simulink model "s_function_model"  (R2021b)
settings: Solver=FixedStepAuto  StartTime=0.0  StopTime=10.0  RelTol=1e-3
settings Model: Creator=krzysztof  LastModifiedBy=krzysztof
settings SolverCC: ZeroCrossControl=DisableAll
settings DataIOCC: SaveOutput=off  SaveTime=off
settings OptimizationCC: BlockReduction=off  DefaultParameterBehavior=Inlined

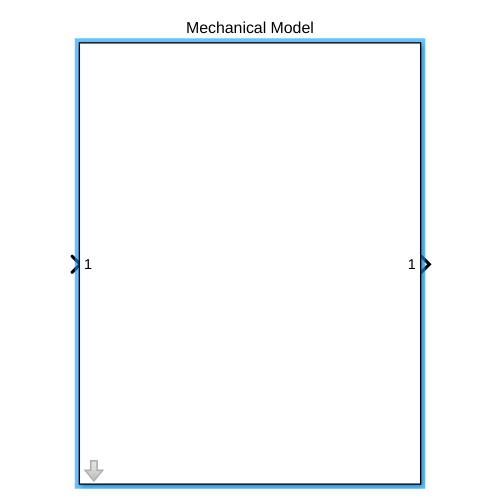
[thumbnail: Simulink's stored preview of the top-level diagram]
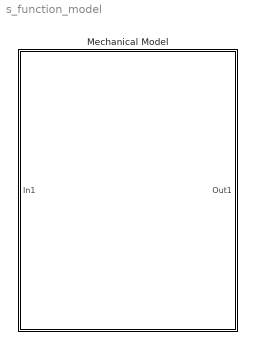
== system s_function_model ==
  Mechanical Model : Subsystem
      mask help: Simulink:masks:GenSFuncDesc_MD
      mask Help: eval('feval(''rtwprivate'',''rtwhelpview'',''rtw_sfcn_block'')');

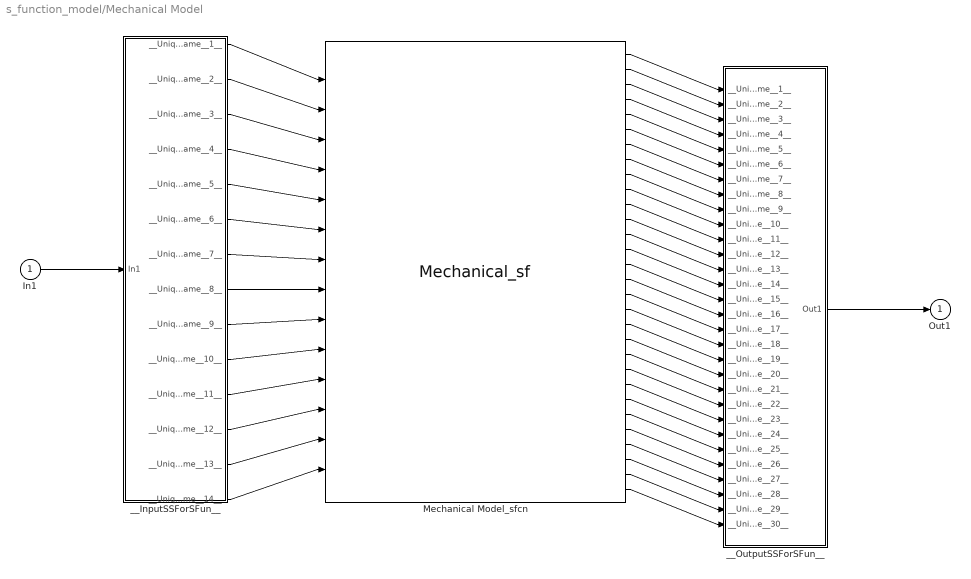
== system s_function_model/Mechanical Model ==
  In1 : Inport
  Mechanical Model_sfcn : S-Function  FunctionName=Mechanical_sf  SFunctionModules=""  SFunctionDeploymentMode=off  EnableBusSupport=off  mask{rtw_sf_name=Mechanical_sf, showVar=off}
      mask prompts: rtw_sf_name "Simulink:masks:GenSFuncName_MP"; showVar "Simulink:masks:GenSFuncShowModuleList_MP"
      mask help: Simulink:masks:GenSFuncDesc_MD
      mask init:
      | displist = '';
      | if ~strcmp(get_param(gcb, 'FunctionName'), rtw_sf_name);
      |   set_param(gcb, 'FunctionName', rtw_sf_name);
      | end
      | % Check if we are generating code
      | rtw_mode = false;
      | if strcmpi(get_param(bdroot(gcb),'SimulationStatus'),'Initializing')
      | 	rtw_mode = strcmpi(get_param(bdroot(gcb),'BuildingRTWCode'),'on') && ...
      | 		~strcmpi(get_param(bdroot(gcb),'TargetStyle'),'SimulationTarget');
      | end
      | if showVar || rtw_mode
      | 	if exist('rtwsfunc') == 2 | exist('rtwsfunc') == 6
      | 		tmplist = rtwsfunc(rtw_sf_name,gcb);
      | 		tmplist = DAStudio.message('Simulink:masks:GenSFuncListOfModules_IC', tmplist);
      | 	elseif showVar
      | 		tmplist1 = DAStudio.message('Simulink:masks:GenSFuncListOfModules_IC', '');
      |         tmplist2 = DAStudio.message('Simulink:masks:GenSFuncNotLicensed_IC');
      |         tmplist = [tmplist1 tmplist2];
      |  	end
      | end
      | if showVar
      |   displist = tmplist;
      | end
      settings: CopyFcn=|
      | if ~strcmp(get_param(gcb,'Linkstatus'),'none') && ...
      | ~strcmp(get_param(gcb,'Linkstatus'),'implicit')
      |   set_param(gcb,'LinkStatus','none');
      | end
      mask Help: eval('feval(''rtwprivate'',''rtwhelpview'',''rtw_sfcn_block'')');
      mask Display:
      | port_label('input',1,'u');
      | port_label('input',2,'d');
      | port_label('input',3,'p');
      | port_label('input',4,'m_mass');
      | port_label('input',5,'m_platf');
      | port_label('input',6,'J_platf');
      | port_label('input',7,'roff');
      | port_label('input',8,'g');
      | port_label('input',9,'tau');
      | port_label('input',10,'w0');
      | port_label('input',11,'q0');
      | port_label('input',12,'umax');
      | port_label('input',13,'signal13');
      | port_label('input',14,'debug_model');
      | port_label('output',1,'w');
      | port_label('output',2,'wg');
      | port_label('output',3,'wp');
      | port_label('output',4,'C');
      | port_label('output',5,'q');
      | port_label('output',6,'angle_between_zw_zb');
      | port_label('output',7,'gb');
      | port_label('output',8,'M');
      | port_label('output',9,'r_COM');
      | port_label('output',10,'r_b');
      | port_label('output',11,'vis_angl_rad');
      | port_label('output',12,'H');
      | port_label('output',13,'Hdot_minus1');
      | port_label('output',14,'J_masses');
      | port_label('output',15,'etot');
      | port_label('output',16,'ekin');
      | port_label('output',17,'epot');
      | port_label('output',18,'epot_outside');
      | port_label('output',19,'ub');
      | port_label('output',20,'db');
      | port_label('output',21,'pb');
      | port_label('output',22,'m_massb');
      | port_label('output',23,'m_platfb');
      | port_label('output',24,'J_platfb');
      | port_label('output',25,'roffb');
      | port_label('output',26,'taub');
      | port_label('output',27,'ga');
      | port_label('output',28,'w0b');
      | port_label('output',29,'q0b');
      | port_label('output',30,'umaxb');
  __InputSSForSFun__ : Subsystem
  __OutputSSForSFun__ : Subsystem
  Out1 : Outport
  wires:
  In1/1 -> __InputSSForSFun__/1(In1)
  __InputSSForSFun__/1(__UniqueOutportName__1__) -> Mechanical Model_sfcn/1
  __InputSSForSFun__/2(__UniqueOutportName__2__) -> Mechanical Model_sfcn/2
  __InputSSForSFun__/3(__UniqueOutportName__3__) -> Mechanical Model_sfcn/3
  __InputSSForSFun__/4(__UniqueOutportName__4__) -> Mechanical Model_sfcn/4
  __InputSSForSFun__/5(__UniqueOutportName__5__) -> Mechanical Model_sfcn/5
  __InputSSForSFun__/6(__UniqueOutportName__6__) -> Mechanical Model_sfcn/6
  __InputSSForSFun__/7(__UniqueOutportName__7__) -> Mechanical Model_sfcn/7
  __InputSSForSFun__/8(__UniqueOutportName__8__) -> Mechanical Model_sfcn/8
  __InputSSForSFun__/9(__UniqueOutportName__9__) -> Mechanical Model_sfcn/9
  __InputSSForSFun__/10(__UniqueOutportName__10__) -> Mechanical Model_sfcn/10
  __InputSSForSFun__/11(__UniqueOutportName__11__) -> Mechanical Model_sfcn/11
  __InputSSForSFun__/12(__UniqueOutportName__12__) -> Mechanical Model_sfcn/12
  __InputSSForSFun__/13(__UniqueOutportName__13__) -> Mechanical Model_sfcn/13
  __InputSSForSFun__/14(__UniqueOutportName__14__) -> Mechanical Model_sfcn/14
  Mechanical Model_sfcn/1 -> __OutputSSForSFun__/1(__UniqueInportName__1__)
  Mechanical Model_sfcn/2 -> __OutputSSForSFun__/2(__UniqueInportName__2__)
  Mechanical Model_sfcn/3 -> __OutputSSForSFun__/3(__UniqueInportName__3__)
  Mechanical Model_sfcn/4 -> __OutputSSForSFun__/4(__UniqueInportName__4__)
  Mechanical Model_sfcn/5 -> __OutputSSForSFun__/5(__UniqueInportName__5__)
  Mechanical Model_sfcn/6 -> __OutputSSForSFun__/6(__UniqueInportName__6__)
  Mechanical Model_sfcn/7 -> __OutputSSForSFun__/7(__UniqueInportName__7__)
  Mechanical Model_sfcn/8 -> __OutputSSForSFun__/8(__UniqueInportName__8__)
  Mechanical Model_sfcn/9 -> __OutputSSForSFun__/9(__UniqueInportName__9__)
  Mechanical Model_sfcn/10 -> __OutputSSForSFun__/10(__UniqueInportName__10__)
  Mechanical Model_sfcn/11 -> __OutputSSForSFun__/11(__UniqueInportName__11__)
  Mechanical Model_sfcn/12 -> __OutputSSForSFun__/12(__UniqueInportName__12__)
  Mechanical Model_sfcn/13 -> __OutputSSForSFun__/13(__UniqueInportName__13__)
  Mechanical Model_sfcn/14 -> __OutputSSForSFun__/14(__UniqueInportName__14__)
  Mechanical Model_sfcn/15 -> __OutputSSForSFun__/15(__UniqueInportName__15__)
  Mechanical Model_sfcn/16 -> __OutputSSForSFun__/16(__UniqueInportName__16__)
  Mechanical Model_sfcn/17 -> __OutputSSForSFun__/17(__UniqueInportName__17__)
  Mechanical Model_sfcn/18 -> __OutputSSForSFun__/18(__UniqueInportName__18__)
  Mechanical Model_sfcn/19 -> __OutputSSForSFun__/19(__UniqueInportName__19__)
  Mechanical Model_sfcn/20 -> __OutputSSForSFun__/20(__UniqueInportName__20__)
  Mechanical Model_sfcn/21 -> __OutputSSForSFun__/21(__UniqueInportName__21__)
  Mechanical Model_sfcn/22 -> __OutputSSForSFun__/22(__UniqueInportName__22__)
  Mechanical Model_sfcn/23 -> __OutputSSForSFun__/23(__UniqueInportName__23__)
  Mechanical Model_sfcn/24 -> __OutputSSForSFun__/24(__UniqueInportName__24__)
  Mechanical Model_sfcn/25 -> __OutputSSForSFun__/25(__UniqueInportName__25__)
  Mechanical Model_sfcn/26 -> __OutputSSForSFun__/26(__UniqueInportName__26__)
  Mechanical Model_sfcn/27 -> __OutputSSForSFun__/27(__UniqueInportName__27__)
  Mechanical Model_sfcn/28 -> __OutputSSForSFun__/28(__UniqueInportName__28__)
  Mechanical Model_sfcn/29 -> __OutputSSForSFun__/29(__UniqueInportName__29__)
  Mechanical Model_sfcn/30 -> __OutputSSForSFun__/30(__UniqueInportName__30__)
  __OutputSSForSFun__/1(Out1) -> Out1/1

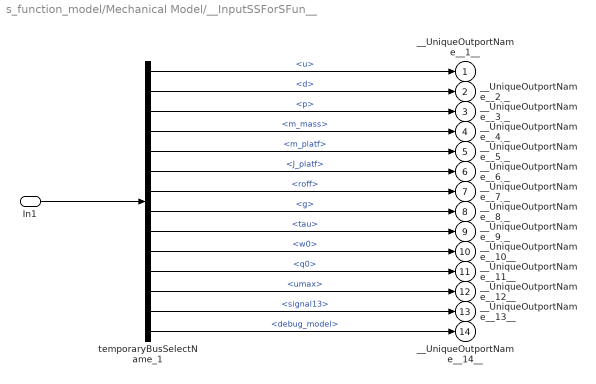
== system s_function_model/Mechanical Model/__InputSSForSFun__ ==
  In1 : Inport
  temporaryBusSelectName_1 : BusSelector  OutputSignals=u,d,p,m_mass,m_platf,J_platf,roff,g,tau,w0,q0,umax,signal13,debug_model
  __UniqueOutportName__1__ : Outport
  __UniqueOutportName__2__ : Outport  Port=2
  __UniqueOutportName__3__ : Outport  Port=3
  __UniqueOutportName__4__ : Outport  Port=4
  __UniqueOutportName__5__ : Outport  Port=5
  __UniqueOutportName__6__ : Outport  Port=6
  __UniqueOutportName__7__ : Outport  Port=7
  __UniqueOutportName__8__ : Outport  Port=8
  __UniqueOutportName__9__ : Outport  Port=9
  __UniqueOutportName__10__ : Outport  Port=10
  __UniqueOutportName__11__ : Outport  Port=11
  __UniqueOutportName__12__ : Outport  Port=12
  __UniqueOutportName__13__ : Outport  Port=13
  __UniqueOutportName__14__ : Outport  Port=14
  wires:
  In1/1 -> temporaryBusSelectName_1/1
  temporaryBusSelectName_1/1 -> __UniqueOutportName__1__/1  "<u>"
  temporaryBusSelectName_1/2 -> __UniqueOutportName__2__/1  "<d>"
  temporaryBusSelectName_1/3 -> __UniqueOutportName__3__/1  "<p>"
  temporaryBusSelectName_1/4 -> __UniqueOutportName__4__/1  "<m_mass>"
  temporaryBusSelectName_1/5 -> __UniqueOutportName__5__/1  "<m_platf>"
  temporaryBusSelectName_1/6 -> __UniqueOutportName__6__/1  "<J_platf>"
  temporaryBusSelectName_1/7 -> __UniqueOutportName__7__/1  "<roff>"
  temporaryBusSelectName_1/8 -> __UniqueOutportName__8__/1  "<g>"
  temporaryBusSelectName_1/9 -> __UniqueOutportName__9__/1  "<tau>"
  temporaryBusSelectName_1/10 -> __UniqueOutportName__10__/1  "<w0>"
  temporaryBusSelectName_1/11 -> __UniqueOutportName__11__/1  "<q0>"
  temporaryBusSelectName_1/12 -> __UniqueOutportName__12__/1  "<umax>"
  temporaryBusSelectName_1/13 -> __UniqueOutportName__13__/1  "<signal13>"
  temporaryBusSelectName_1/14 -> __UniqueOutportName__14__/1  "<debug_model>"

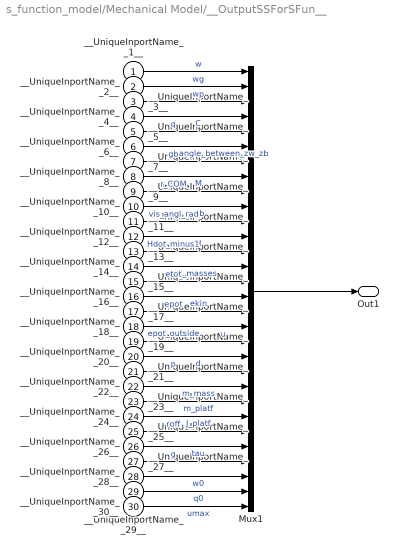
== system s_function_model/Mechanical Model/__OutputSSForSFun__ ==
  __UniqueInportName__1__ : Inport
  __UniqueInportName__2__ : Inport  Port=2
  __UniqueInportName__3__ : Inport  Port=3
  __UniqueInportName__4__ : Inport  Port=4
  __UniqueInportName__5__ : Inport  Port=5
  __UniqueInportName__6__ : Inport  Port=6
  __UniqueInportName__7__ : Inport  Port=7
  __UniqueInportName__8__ : Inport  Port=8
  __UniqueInportName__9__ : Inport  Port=9
  __UniqueInportName__10__ : Inport  Port=10
  __UniqueInportName__11__ : Inport  Port=11
  __UniqueInportName__12__ : Inport  Port=12
  __UniqueInportName__13__ : Inport  Port=13
  __UniqueInportName__14__ : Inport  Port=14
  __UniqueInportName__15__ : Inport  Port=15
  __UniqueInportName__16__ : Inport  Port=16
  __UniqueInportName__17__ : Inport  Port=17
  __UniqueInportName__18__ : Inport  Port=18
  __UniqueInportName__19__ : Inport  Port=19
  __UniqueInportName__20__ : Inport  Port=20
  __UniqueInportName__21__ : Inport  Port=21
  __UniqueInportName__22__ : Inport  Port=22
  __UniqueInportName__23__ : Inport  Port=23
  __UniqueInportName__24__ : Inport  Port=24
  __UniqueInportName__25__ : Inport  Port=25
  __UniqueInportName__26__ : Inport  Port=26
  __UniqueInportName__27__ : Inport  Port=27
  __UniqueInportName__28__ : Inport  Port=28
  __UniqueInportName__29__ : Inport  Port=29
  __UniqueInportName__30__ : Inport  Port=30
  Mux1 : BusCreator  Inputs=30
  Out1 : Outport
  wires:
  __UniqueInportName__1__/1 -> Mux1/1  "w"
  __UniqueInportName__2__/1 -> Mux1/2  "wg"
  __UniqueInportName__3__/1 -> Mux1/3  "wp"
  __UniqueInportName__4__/1 -> Mux1/4  "C"
  __UniqueInportName__5__/1 -> Mux1/5  "q"
  __UniqueInportName__6__/1 -> Mux1/6  "angle_between_zw_zb"
  __UniqueInportName__7__/1 -> Mux1/7  "gb"
  __UniqueInportName__8__/1 -> Mux1/8  "M"
  __UniqueInportName__9__/1 -> Mux1/9  "r_COM"
  __UniqueInportName__10__/1 -> Mux1/10  "r_b"
  __UniqueInportName__11__/1 -> Mux1/11  "vis_angl_rad"
  __UniqueInportName__12__/1 -> Mux1/12  "H"
  __UniqueInportName__13__/1 -> Mux1/13  "Hdot_minus1"
  __UniqueInportName__14__/1 -> Mux1/14  "J_masses"
  __UniqueInportName__15__/1 -> Mux1/15  "etot"
  __UniqueInportName__16__/1 -> Mux1/16  "ekin"
  __UniqueInportName__17__/1 -> Mux1/17  "epot"
  __UniqueInportName__18__/1 -> Mux1/18  "epot_outside"
  __UniqueInportName__19__/1 -> Mux1/19  "u"
  __UniqueInportName__20__/1 -> Mux1/20  "d"
  __UniqueInportName__21__/1 -> Mux1/21  "p"
  __UniqueInportName__22__/1 -> Mux1/22  "m_mass"
  __UniqueInportName__23__/1 -> Mux1/23  "m_platf"
  __UniqueInportName__24__/1 -> Mux1/24  "J_platf"
  __UniqueInportName__25__/1 -> Mux1/25  "roff"
  __UniqueInportName__26__/1 -> Mux1/26  "tau"
  __UniqueInportName__27__/1 -> Mux1/27  "g"
  __UniqueInportName__28__/1 -> Mux1/28  "w0"
  __UniqueInportName__29__/1 -> Mux1/29  "q0"
  __UniqueInportName__30__/1 -> Mux1/30  "umax"
  Mux1/1 -> Out1/1
